simulink model "controller"  (R2022a)
settings: Solver=FixedStepAuto  StartTime=0.0  StopTime=10.0  FixedStep=1/10  RelTol=1e-3
libraries: simulink x1
settings Model: Creator=DAUIN-Win10  LastModifiedBy=alexf
settings DebuggingCC: UnconnectedInputMsg=warning  UnconnectedOutputMsg=warning  UnconnectedLineMsg=warning
settings RTWCC: DLArmComputeVersion=19.05

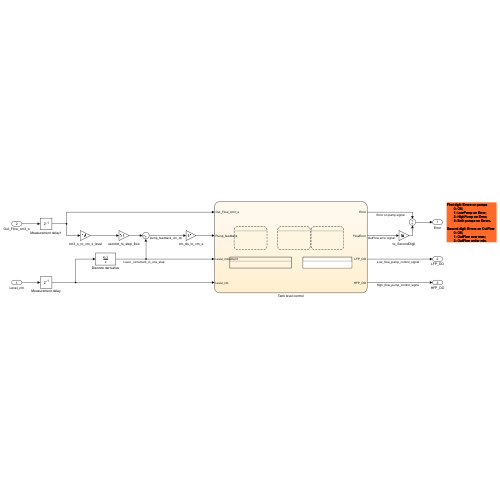
[thumbnail: Simulink's stored preview of the top-level diagram]
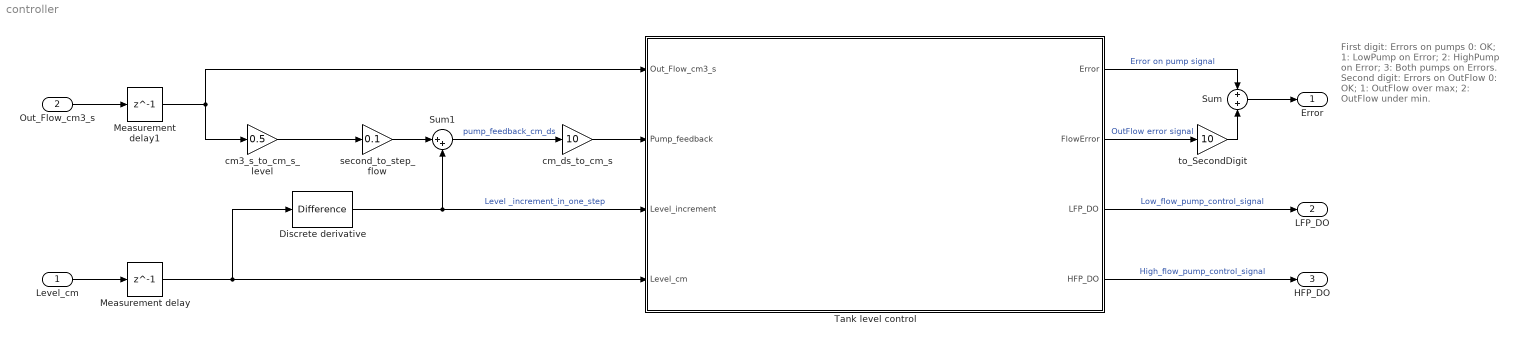
== system controller ==
  note: First digit: Errors on pumps
      | 0: OK;
      | 1: LowPump on Error;
      | 2: HighPump on Error;
      | 3: Both pumps on Errors.
      |
      | Second digit: Errors on OutFlow
      | 0: OK;
      | 1: OutFlow over max;
      | 2: OutFlow under min.
  Level_cm : Inport  OutDataTypeStr=double
  Out_Flow_cm3_s : Inport  Port=2  OutDataTypeStr=double
  Discrete derivative : simulink/Discrete/Difference  ICPrevInput=0.0  OutMin=[]  OutMax=[]  OutDataType=fixdt(1, 16)  OutScaling=2^-10  DoSatur=off
  Measurement delay : Delay  DelayLength=1
  Measurement delay1 : Delay  DelayLength=1
  Sum : Sum  Inputs=+|+  AccumDataTypeStr=uint8
  Sum1 : Sum  Inputs=|++
  Tank level control : Stateflow chart  TreatAsAtomicUnit=on
  cm3_s_to_cm_s_level : Gain  Gain=0.5
  cm_ds_to_cm_s : Gain  Gain=10
  second_to_step_flow : Gain  Gain=0.1
  to_SecondDigit : Gain  Gain=10  ParamDataTypeStr=uint8  OutDataTypeStr=uint8  SaturateOnIntegerOverflow=on
  Error : Outport  OutDataTypeStr=uint8
  LFP_DO : Outport  Port=2  OutDataTypeStr=boolean
  HFP_DO : Outport  Port=3  OutDataTypeStr=boolean
  wires:
  Level_cm/1 -> Measurement delay/1
  Measurement delay/1 -> Tank level control/4(Level_cm), Discrete derivative/1
  Tank level control/1(Error) -> Sum/1  "Error on pump signal"
  Discrete derivative/1 -> Sum1/2, Tank level control/3(Level_increment)  "Level _increment_in_one_step"
  cm3_s_to_cm_s_level/1 -> second_to_step_flow/1
  second_to_step_flow/1 -> Sum1/1
  Sum1/1 -> cm_ds_to_cm_s/1  "pump_feedback_cm_ds"
  cm_ds_to_cm_s/1 -> Tank level control/2(Pump_feedback)
  Out_Flow_cm3_s/1 -> Measurement delay1/1
  Tank level control/3(LFP_DO) -> LFP_DO/1  "Low_flow_pump_control_signal"
  Tank level control/4(HFP_DO) -> HFP_DO/1  "High_flow_pump_control_signal"
  Tank level control/2(FlowError) -> to_SecondDigit/1  "OutFlow error signal"
  to_SecondDigit/1 -> Sum/2
  Sum/1 -> Error/1
  Measurement delay1/1 -> cm3_s_to_cm_s_level/1, Tank level control/1(Out_Flow_cm3_s)

== stateflow chart controller/Tank level control ==
  state PumpLogic [parallel]
    during: PumpTable(isFilling(Level_increment), Level_cm);
    settings: executionOrder=1
    (history)
    state PumpOff
      en:
      LFP_DO=0;
      HFP_DO=0;
    state PumpLo
      en:
      LFP_DO=1;
      HFP_DO=0;
    state PumpHi
      en:
      LFP_DO=0;
      HFP_DO=1;
    note: In case of fault of one of the two pumps, the other pump will be used as backup
    (default) -> PumpOff
    PumpOff -> PumpLo [order 1] : [(pump_mode==1 && Error!=1 && Error!=3) || (pump_mode==2&&Error==2)]
    PumpLo -> PumpOff [order 1] : [pump_mode==0 || Error==3]
    (junction 38) -> PumpOff
    (junction 36) -> PumpLo
    PumpOff -> (junction 34) [order 2] : [(pump_mode==2 && Error!=2 && Error!=3) || (pump_mode==1 && Error==1 && Error!=3)]
    PumpLo -> (junction 41) [order 2] : [pump_mode==2 && Error!=2 && Error!=3 || (pump_mode==1 && Error==1)]
    PumpHi -> (junction 36) [order 1] : [(pump_mode==1 && Error!=1 && Error!=3) || (pump_mode==2 && Error==2)]
    (junction 34) -> PumpHi
    (junction 41) -> PumpHi
    PumpHi -> (junction 38) [order 2] : [pump_mode==0 || Error==3]
  state ErrorLogic [parallel]
    settings: executionOrder=2
    state OK
      Error=0;
    state WarningLFP
      en: i=i+1;
    state LFPerror
      Error=1;
    state WarningHFP
      en: i=i+1;
    state WarningHFPandLFPerror
      en: i=i+1;
    state HFPerror
      Error=2;
    state WarningLFPandHFPerror
      en: i=i+1;
    state PumpsError
      Error=3;
    (default) -> OK
    OK -> WarningLFP [order 1] : [LFP_DO==1 && (Pump_feedback<0.9 || Pump_feedback>1.1)]
        | {i=0;}
    WarningLFP -> (junction 197) [order 3] : [LFP_DO==1 && (Pump_feedback<0.9 || Pump_feedback>1.1)]
    (junction 197) -> (junction 198)
    WarningLFP -> OK [order 2] : [(LFP_DO==1 && (Pump_feedback>0.9 &&Pump_feedback<1.1))]
        | {i=0}
    (junction 233) -> WarningLFP
    (junction 198) -> WarningLFP
    (junction 232) -> (junction 233)
    WarningLFP -> (junction 236) [order 4] : [HFP_DO==1 && (Pump_feedback<2.7||Pump_feedback>3.3)]
        | {i=0;}
    (junction 236) -> (junction 237)
    OK -> WarningHFP [order 2] : [HFP_DO==1 && (Pump_feedback<2.7||Pump_feedback>3.3)]
        | {i=0;}
    WarningHFP -> OK [order 2] : [(HFP_DO==1 && (Pump_feedback>2.7&&Pump_feedback<3.3)) || HFP_DO==0]
        | {i=0;}
    WarningLFP -> LFPerror [order 1] : [i==5]
    WarningHFP -> (junction 221) [order 4] : [HFP_DO==1 && (Pump_feedback<2.7||Pump_feedback>3.3)]
    WarningHFP -> (junction 232) [order 3] : [LFP_DO==1 && (Pump_feedback<0.9 || Pump_feedback>1.1)]
        | {i=0;}
    (junction 221) -> (junction 222)
    WarningHFPandLFPerror -> LFPerror [order 2] : [HFP_DO==1 && (Pump_feedback>2.7&&Pump_feedback<3.3)]
    LFPerror -> WarningHFPandLFPerror : [(HFP_DO==1 && (Pump_feedback<2.7||Pump_feedback>3.3)) || HFP_DO==0]
        | {i=0;}
    (junction 222) -> WarningHFP
    (junction 237) -> WarningHFP
    WarningHFP -> HFPerror [order 1] : [i==5]
    WarningHFPandLFPerror -> (junction 205) [order 3] : [HFP_DO==1 && (Pump_feedback<2.7||Pump_feedback>3.3)]
    (junction 205) -> (junction 206)
    (junction 206) -> WarningHFPandLFPerror
    HFPerror -> WarningLFPandHFPerror : [LFP_DO==1 && (Pump_feedback<0.9 || Pump_feedback>1.1)]
        | {i=0;}
    WarningLFPandHFPerror -> HFPerror [order 2] : [LFP_DO==1 && (Pump_feedback>0.9&&Pump_feedback<1.1)]
        | {i=0;}
    WarningHFPandLFPerror -> PumpsError [order 1] : [i==5]
    WarningLFPandHFPerror -> (junction 230) [order 3] : [LFP_DO==1 && (Pump_feedback<0.9 || Pump_feedback>1.1)]
    (junction 230) -> (junction 226)
    WarningLFPandHFPerror -> PumpsError [order 1] : [i==5]
    (junction 226) -> WarningLFPandHFPerror
  state AdditionalErrorLogic [parallel]
    settings: executionOrder=3
    state OutFlowLimitsErrorLogic [parallel]
      settings: executionOrder=1
      state OutFlowInLimits
        en: FlowError=0;
      state OutFlowOverMaximum
        en: FlowError=1;
      state OutFlowUnderMinimum
        en: FlowError=2;
      (default) -> OutFlowInLimits
      OutFlowInLimits -> OutFlowOverMaximum [order 1] : [Out_Flow_cm3_s > 1]
      OutFlowOverMaximum -> OutFlowInLimits : [Out_Flow_cm3_s<1]
      OutFlowUnderMinimum -> OutFlowInLimits : [Out_Flow_cm3_s>0.5]
      OutFlowInLimits -> OutFlowUnderMinimum [order 2] : [Out_Flow_cm3_s<0.5]
    state DoublePumpErrorLogic [parallel]
      settings: executionOrder=2
      state SinglePump
      state DoublePumpError
        en: HFP_DO = 0;
      (default) -> SinglePump
      DoublePumpError -> SinglePump
      SinglePump -> DoublePumpError : [LFP_DO == 1 && HFP_DO == 1]
  state status = isFilling(increment) [function]
    (default) -> (junction 74)
    (junction 74) -> (junction 78) [order 1] : [increment>0]
    (junction 74) -> (junction 79) [order 2] : {status=0;}
    (junction 78) -> (junction 82) : {status=1;}
    (junction 82) -> (junction 79)
    (junction 79) -> (junction 86)
  state PumpTable(filling, level) [function]
    (default) -> (junction 96)
    (junction 96) -> (junction 98) : {
        | /* The level is increasing */
        | aVarTruthTableCondition_1 = (filling == 1);
        | }
    (junction 98) -> (junction 100) : {
        | /* The level is below 150cm */
        | aVarTruthTableCondition_2 = (level < 150);
        | }
    (junction 100) -> (junction 102) : {
        | /* The level is below 175cm */
        | aVarTruthTableCondition_3 = (level < 175);
        | }
    (junction 102) -> (junction 104) : {
        | /* The level is over 180cm */
        | aVarTruthTableCondition_4 = (level > 180);
        | }
    (junction 104) -> (junction 106) : {
        | /* The level is over 155cm */
        | aVarTruthTableCondition_5 = (level > 155);
        | }
    (junction 106) -> (junction 108) [order 1] : [!aVarTruthTableCondition_1 && aVarTruthTableCondition_2]
    (junction 108) -> (junction 110) : {
        | /* 'A3':Low pump off High pump on */
        | pump_mode = 2;
        | }
    (junction 106) -> (junction 112) [order 2]
    (junction 112) -> (junction 114) [order 1] : [!aVarTruthTableCondition_1 && !aVarTruthTableCondition_2 && aVarTruthTableCondition_3]
    (junction 114) -> (junction 116) : {
        | /* 'A2':Low pump on High pump off */
        | pump_mode = 1;
        | }
    (junction 112) -> (junction 118) [order 2]
    (junction 118) -> (junction 120) [order 1] : [aVarTruthTableCondition_1 && !aVarTruthTableCondition_4 && aVarTruthTableCondition_5]
    (junction 120) -> (junction 122) : {
        | /* 'A2':Low pump on High pump off */
        | pump_mode = 1;
        | }
    (junction 118) -> (junction 124) [order 2]
    (junction 124) -> (junction 126) [order 1] : [aVarTruthTableCondition_1 && aVarTruthTableCondition_4]
    (junction 126) -> (junction 128) : {
        | /* 'A1':Pumps off */
        | pump_mode = 0;
        | }
    (junction 124) -> (junction 178) [order 2]
    (junction 178) -> (junction 180) : /* Default */
    (junction 180) -> (junction 265) : {
        | /* 'A4':Pump mode remain inalterate */
        | pump_mode = pump_mode;
        | }
  data: increment function_input double; status function_output double; filling function_input double; level function_input double; aVarTruthTableCondition_1 temporary boolean =0; aVarTruthTableCondition_2 temporary boolean =0; aVarTruthTableCondition_3 temporary boolean =0; aVarTruthTableCondition_4 temporary boolean =0; aVarTruthTableCondition_5 temporary boolean =0; Out_Flow_cm3_s input; Pump_feedback input; Level_increment input; Error output uint8; FlowError output uint8; Level_cm input double size=1; LFP_DO output boolean size=1; HFP_DO output boolean size=1; pump_mode local uint8; i local int64
  data aVarTruthTableCondition_1 settings: description=The level is increasing
  data aVarTruthTableCondition_2 settings: description=The level is below 150cm
  data aVarTruthTableCondition_3 settings: description=The level is below 175cm
  data aVarTruthTableCondition_4 settings: description=The level is over 180cm
  data aVarTruthTableCondition_5 settings: description=The level is over 155cm
